simulink model "quad"  (R2022a)
settings: Solver=VariableStepAuto  StartTime=0.0  StopTime=5  RelTol=1e-3
values from neighbouring files (symbols this model uses):
  kp_yaw = omega_n_yaw^2*Izc    (= 0.0175335533676)    [ParamsInit_test.m]
undefined symbols (not defined in the file or in its folder): kp_height, kp_pitch, kp_roll, ModelInit_RPM, ModelParam_motorT, Newton, Raphson, stateInp, Timestep, Vehicle
libraries: simulink_extras x3, shared6dof x1
settings Model: Creator=Admin  LastModifiedBy=gaowe
settings SolverCC: AlgebraicLoopSolver=TrustRegion
settings DebuggingCC: UnconnectedInputMsg=warning  UnconnectedOutputMsg=warning  UnconnectedLineMsg=warning
settings RTWCC: DLArmComputeVersion=19.05

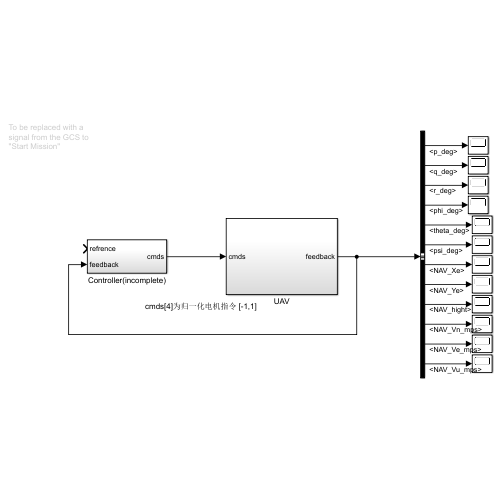
[thumbnail: Simulink's stored preview of the top-level diagram]
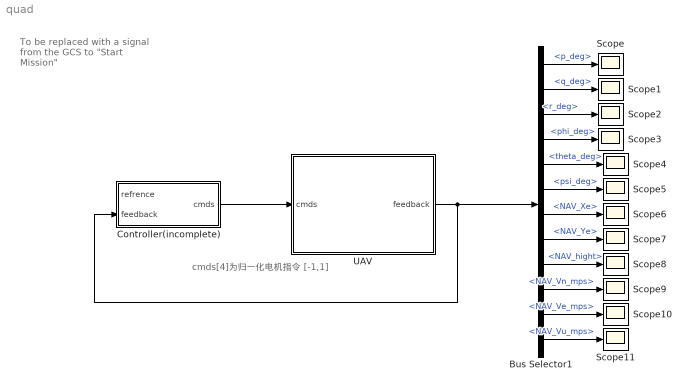
== system quad ==
  note: cmds[4]为归一化电机指令 [-1,1]
  note: To be replaced with a signal from the GCS to "Start Mission"
  Bus Selector1 : BusSelector  OutputSignals=MAG3.p_deg,MAG3.q_deg,MAG3.r_deg,MIDG.phi_deg,MIDG.theta_deg,MIDG.psi_deg,MIDG.NAV_Xe,MIDG.NAV_Ye,MIDG.NAV_hight,MIDG.NAV_Vn_mps,MIDG.NAV_Ve_mps,MIDG.NAV_Vu_mps
  Controller(incomplete) : Subsystem
  Scope{,1..11} (12 alike) : Scope
  UAV : Subsystem
  wires:
  Controller(incomplete)/1(cmds) -> UAV/1(cmds)
  UAV/1(feedback) -> Controller(incomplete)/2(feedback), Bus Selector1/1
  Bus Selector1/1 -> Scope/1  "<p_deg>"
  Bus Selector1/2 -> Scope1/1  "<q_deg>"
  Bus Selector1/3 -> Scope2/1  "<r_deg>"
  Bus Selector1/4 -> Scope3/1  "<phi_deg>"
  Bus Selector1/5 -> Scope4/1  "<theta_deg>"
  Bus Selector1/6 -> Scope5/1  "<psi_deg>"
  Bus Selector1/7 -> Scope6/1  "<NAV_Xe>"
  Bus Selector1/8 -> Scope7/1  "<NAV_Ye>"
  Bus Selector1/9 -> Scope8/1  "<NAV_hight>"
  Bus Selector1/10 -> Scope9/1  "<NAV_Vn_mps>"
  Bus Selector1/11 -> Scope10/1  "<NAV_Ve_mps>"
  Bus Selector1/12 -> Scope11/1  "<NAV_Vu_mps>"

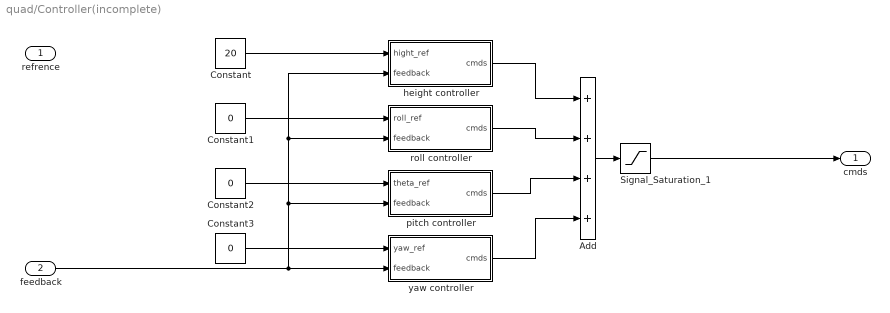
== system quad/Controller(incomplete) ==
  refrence : Inport
  feedback : Inport  Port=2
  Add : Sum  Inputs=++++
  Constant : Constant  Value=20
  Constant1 : Constant  Value=0
  Constant2 : Constant  Value=0
  Constant3 : Constant  Value=0
  Signal_Saturation_1 : Saturate  UpperLimit=[1 1 1 1]  LowerLimit=[-1 -1 -1 -1]
  height controller : Subsystem
  pitch controller : Subsystem
  roll controller : Subsystem
  yaw controller : Subsystem
  cmds : Outport
  wires:
  feedback/1 -> yaw controller/2(feedback), height controller/2(feedback), roll controller/2(feedback), pitch controller/2(feedback)
  Constant/1 -> height controller/1(hight_ref)
  Constant1/1 -> roll controller/1(roll_ref)
  roll controller/1(cmds) -> Add/2
  pitch controller/1(cmds) -> Add/3
  yaw controller/1(cmds) -> Add/4
  height controller/1(cmds) -> Add/1
  Add/1 -> Signal_Saturation_1/1
  Constant2/1 -> pitch controller/1(theta_ref)
  Constant3/1 -> yaw controller/1(yaw_ref)
  Signal_Saturation_1/1 -> cmds/1

== system quad/UAV ==
  cmds : Inport
  FM : Subsystem
  Sensors : Subsystem
  UAV Model : Subsystem
  feedback : Outport
  wires:
  UAV Model/2(Aux_Vars) -> Sensors/2(Aux_Vars), FM/3(Aux_Vars)
  FM/1(F_cg) -> UAV Model/1(Forces)
  FM/2(M_cg) -> UAV Model/2(Moments)
  UAV Model/1(EOM_States) -> Sensors/1(EOM_States), FM/2(EOM_States)
  Sensors/1(sensors) -> feedback/1
  cmds/1 -> FM/1(cmds)

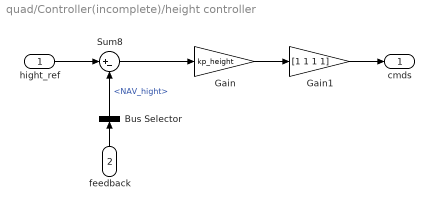
== system quad/Controller(incomplete)/height controller ==
  hight_ref : Inport
  feedback : Inport  Port=2
  Bus Selector : BusSelector  OutputSignals=MIDG.NAV_hight
  Gain : Gain  Gain=kp_height
  Gain1 : Gain  Gain=[1 1 1 1]
  Sum8 : Sum  Inputs=|+-
  cmds : Outport  VectorParamsAs1DForOutWhenUnconnected=off
  wires:
  hight_ref/1 -> Sum8/1
  feedback/1 -> Bus Selector/1
  Sum8/1 -> Gain/1
  Gain/1 -> Gain1/1
  Bus Selector/1 -> Sum8/2  "<NAV_hight>"
  Gain1/1 -> cmds/1

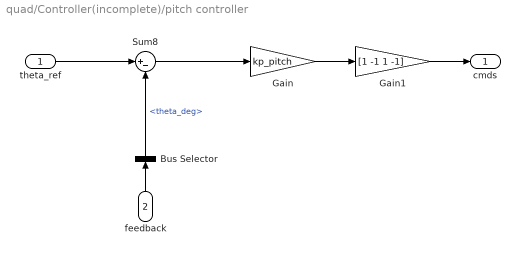
== system quad/Controller(incomplete)/pitch controller ==
  theta_ref : Inport
  feedback : Inport  Port=2
  Bus Selector : BusSelector  OutputSignals=MIDG.theta_deg
  Gain : Gain  Gain=kp_pitch
  Gain1 : Gain  Gain=[1 -1 1 -1]
  Sum8 : Sum  Inputs=|+-
  cmds : Outport  VectorParamsAs1DForOutWhenUnconnected=off
  wires:
  feedback/1 -> Bus Selector/1
  Sum8/1 -> Gain/1
  theta_ref/1 -> Sum8/1
  Gain/1 -> Gain1/1
  Bus Selector/1 -> Sum8/2  "<theta_deg>"
  Gain1/1 -> cmds/1

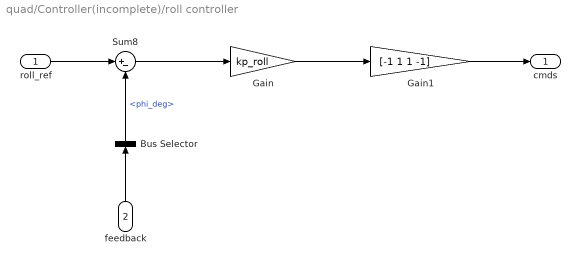
== system quad/Controller(incomplete)/roll controller ==
  roll_ref : Inport
  feedback : Inport  Port=2
  Bus Selector : BusSelector  OutputSignals=MIDG.phi_deg
  Gain : Gain  Gain=kp_roll
  Gain1 : Gain  Gain=[-1 1 1 -1]
  Sum8 : Sum  Inputs=|+-
  cmds : Outport  VectorParamsAs1DForOutWhenUnconnected=off
  wires:
  roll_ref/1 -> Sum8/1
  Sum8/1 -> Gain/1
  feedback/1 -> Bus Selector/1
  Gain/1 -> Gain1/1
  Bus Selector/1 -> Sum8/2  "<phi_deg>"
  Gain1/1 -> cmds/1

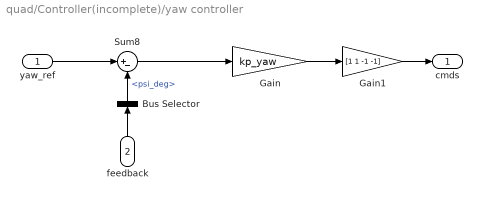
== system quad/Controller(incomplete)/yaw controller ==
  yaw_ref : Inport
  feedback : Inport  Port=2
  Bus Selector : BusSelector  OutputSignals=MIDG.psi_deg
  Gain : Gain  Gain=kp_yaw
  Gain1 : Gain  Gain=[1 1 -1 -1]
  Sum8 : Sum  Inputs=|+-
  cmds : Outport  VectorParamsAs1DForOutWhenUnconnected=off
  wires:
  feedback/1 -> Bus Selector/1
  Sum8/1 -> Gain/1
  yaw_ref/1 -> Sum8/1
  Gain/1 -> Gain1/1
  Bus Selector/1 -> Sum8/2  "<psi_deg>"
  Gain1/1 -> cmds/1

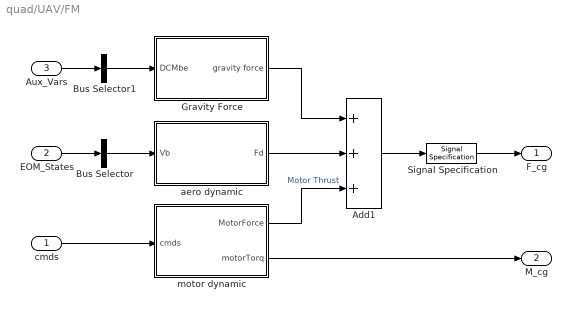
== system quad/UAV/FM ==
  cmds : Inport
  EOM_States : Inport  Port=2  Unit=m/s
  Aux_Vars : Inport  Port=3
  Add1 : Sum  Inputs=+++
  Bus Selector : BusSelector  OutputSignals=ub,wb,vb  OutputAsBus=on
  Bus Selector1 : BusSelector  OutputSignals=DCMbe  OutputAsBus=on
  Gravity Force : Subsystem
  Signal Specification : SignalSpecification  Dimensions=3
  aero dynamic : Subsystem
  motor dynamic : Subsystem
  F_cg : Outport  Unit=N  VectorParamsAs1DForOutWhenUnconnected=off
  M_cg : Outport  Port=2  Unit=N*m  VectorParamsAs1DForOutWhenUnconnected=off
  wires:
  Signal Specification/1 -> F_cg/1
  Aux_Vars/1 -> Bus Selector1/1
  cmds/1 -> motor dynamic/1(cmds)
  motor dynamic/2(motorTorq) -> M_cg/1
  Add1/1 -> Signal Specification/1
  Gravity Force/1(gravity force) -> Add1/1
  motor dynamic/1(MotorForce) -> Add1/3  "Motor Thrust"
  EOM_States/1 -> Bus Selector/1
  aero dynamic/1(Fd) -> Add1/2
  Bus Selector/1 -> aero dynamic/1(Vb)
  Bus Selector1/1 -> Gravity Force/1(DCMbe)

== system quad/UAV/Sensors ==
  EOM_States : Inport
  Aux_Vars : Inport  Port=2
  Bus Creator1 : BusCreator  Inputs=2
  MAG3 IMU : Subsystem
  MIDG II 50 Hz : Subsystem  SystemSampleTime=round(1/Timestep/50)*Timestep
  sensors : Outport
  wires:
  Bus Creator1/1 -> sensors/1
  MIDG II 50 Hz/1(MIDG) -> Bus Creator1/1  "MIDG"
  MAG3 IMU/1(MAG3) -> Bus Creator1/2  "MAG3"
  Aux_Vars/1 -> MIDG II 50 Hz/2(AuxVars)
  EOM_States/1 -> MAG3 IMU/1(EOM_State), MIDG II 50 Hz/1(EOM_State)

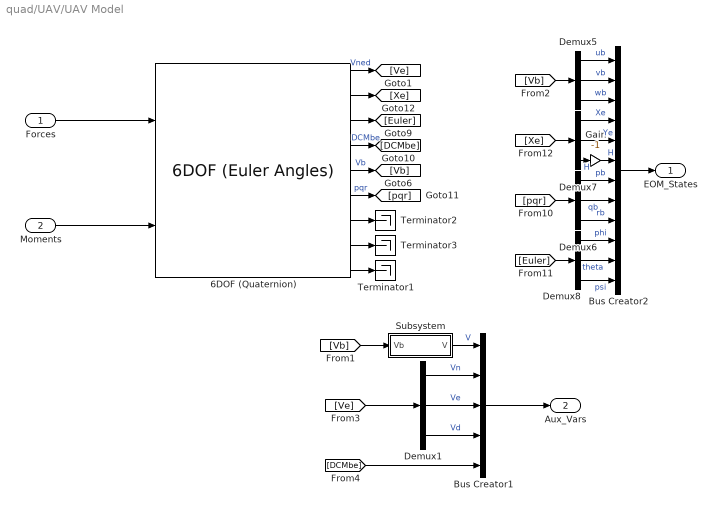
== system quad/UAV/UAV Model ==
  Forces : Inport
  Moments : Inport  Port=2
  6DOF (Quaternion) : shared6dof/6DOF (Euler Angles)  units=Metric (MKS)  mtype=Fixed  rep=Euler Angles  xme_0=stateInp.xyz.*[1 1 -1]  Vm_0=stateInp.uvw  eul_0=stateInp.euler  pm_0=stateInp.pqr  mass_0=Vehicle.Airframe.mass  mass_e=0.5  mass_f=2.0  inertia=Vehicle.Airfame.inertia  inertia_e=eye(3)  inertia_f=2*eye(3)  k_quat=Vehicle.SixDOF.quatGain  vre_flag=on  abi_flag=on  aMode=aMode  xme_statename=''  Vm_statename=''  eul_statename=''  quat_statename=''  pm_statename=''  mass_statename=''
      settings: SourceProductBaseCode=AE,PW,DR,MT,VE
  Bus Creator1 : BusCreator  Inputs=5
  Bus Creator2 : BusCreator  Inputs=12
  Demux{1,5..8} (5 alike) : Demux  Outputs=3
  Gain : Gain  Gain=-1
  Subsystem : Subsystem
  Terminator1 : Terminator
  Terminator2 : Terminator
  Terminator3 : Terminator
  EOM_States : Outport
  Aux_Vars : Outport  Port=2
  wires:
  Moments/1 -> 6DOF (Quaternion)/2
  6DOF (Quaternion)/8 -> Terminator3/1
  6DOF (Quaternion)/7 -> Terminator2/1
  6DOF (Quaternion)/9 -> Terminator1/1
  Forces/1 -> 6DOF (Quaternion)/1
  Demux8/2 -> Bus Creator2/11  "theta"
  [Euler] -> Demux8/1
  [Vb] -> Demux5/1
  Bus Creator2/1 -> EOM_States/1
  [pqr] -> Demux6/1
  Demux6/3 -> Bus Creator2/9  "rb"
  Demux7/1 -> Bus Creator2/4  "Xe"
  [Xe] -> Demux7/1
  Demux7/2 -> Bus Creator2/5  "Ye"
  Demux5/1 -> Bus Creator2/1  "ub"
  Demux6/1 -> Bus Creator2/7  "pb"
  Demux5/2 -> Bus Creator2/2  "vb"
  Demux8/3 -> Bus Creator2/12  "psi"
  Demux7/3 -> Gain/1  "H"
  Demux5/3 -> Bus Creator2/3  "wb"
  Demux8/1 -> Bus Creator2/10  "phi"
  Demux6/2 -> Bus Creator2/8  "qb"
  6DOF (Quaternion)/2 -> [Xe]
  6DOF (Quaternion)/3 -> [Euler]
  6DOF (Quaternion)/4 -> [DCMbe]  "DCMbe"
  6DOF (Quaternion)/5 -> [Vb]  "Vb"
  6DOF (Quaternion)/6 -> [pqr]  "pqr"
  6DOF (Quaternion)/1 -> [Ve]  "Vned"
  Bus Creator1/1 -> Aux_Vars/1
  Subsystem/1(V) -> Bus Creator1/1  "V"
  [Vb] -> Subsystem/1(Vb)
  Demux1/1 -> Bus Creator1/2  "Vn"
  Demux1/2 -> Bus Creator1/3  "Ve"
  Demux1/3 -> Bus Creator1/4  "Vd"
  [Ve] -> Demux1/1
  Gain/1 -> Bus Creator2/6  "H"
  [DCMbe] -> Bus Creator1/5

== system quad/UAV/FM/Gravity Force ==
  DCMbe : Inport
  D2 : Constant  Value=[0 0 9.8]
  Gain1 : Gain  Gain=Vehicle.Airframe.mass
  Product : Product  Multiplication=Matrix(*)
  gravity force : Outport  Unit=N  VectorParamsAs1DForOutWhenUnconnected=off
  wires:
  D2/1 -> Gain1/1
  Gain1/1 -> Product/2  "gravity force NED"
  Product/1 -> gravity force/1
  DCMbe/1 -> Product/1

== system quad/UAV/FM/aero dynamic ==
  Vb : Inport
  Cd : Constant  Value=0.073
  Fd Calculate : MATLAB Function  TreatAsAtomicUnit=on
  Fd : Outport
  wires:
  Cd/1 -> Fd Calculate/2(Cd)
  Fd Calculate/1(Fd) -> Fd/1
  Vb/1 -> Fd Calculate/1(Vb)

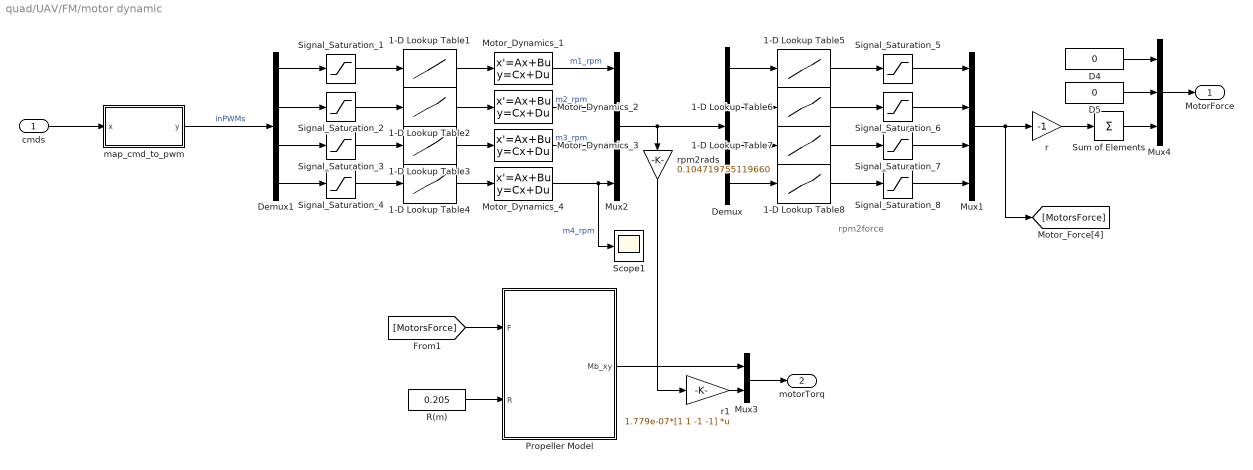
== system quad/UAV/FM/motor dynamic ==
  note: rpm2force
  cmds : Inport
  1-D Lookup Table1 : Lookup_n-D  NumberOfTableDimensions=1  BreakpointsForDimension1=|  BeginIndexSearchUsingPreviousIndexResult=on  Table=|  InternalRulePriority=Speed  RndMeth=Simplest
      BreakpointsForDimension1=|
      | [1301
      | 1347
      | 1402
      | 1459
      | 1522
      | 1591
      | 1661
      | 1702
      | 1778
      | 1932]
      Table=|
      | [2847
      | 3689
      | 4585
      | 5400
      | 6400
      | 7000
      | 7800
      | 8222
      | 9300
      | 10700]
  1-D Lookup Table2 : Lookup_n-D  NumberOfTableDimensions=1  BreakpointsForDimension1=|  BeginIndexSearchUsingPreviousIndexResult=on  Table=|  InternalRulePriority=Speed  RndMeth=Simplest
      BreakpointsForDimension1=|
      | [1301
      | 1347
      | 1402
      | 1459
      | 1522
      | 1591
      | 1661
      | 1702
      | 1778
      | 1932]
      Table=|
      | [2847
      | 3689
      | 4585
      | 5400
      | 6400
      | 7000
      | 7800
      | 8222
      | 9300
      | 10700]
  1-D Lookup Table3 : Lookup_n-D  NumberOfTableDimensions=1  BreakpointsForDimension1=|  BeginIndexSearchUsingPreviousIndexResult=on  Table=|  InternalRulePriority=Speed  RndMeth=Simplest
      BreakpointsForDimension1=|
      | [1301
      | 1347
      | 1402
      | 1459
      | 1522
      | 1591
      | 1661
      | 1702
      | 1778
      | 1932]
      Table=|
      | [2847
      | 3689
      | 4585
      | 5400
      | 6400
      | 7000
      | 7800
      | 8222
      | 9300
      | 10700]
  1-D Lookup Table4 : Lookup_n-D  NumberOfTableDimensions=1  BreakpointsForDimension1=|  BeginIndexSearchUsingPreviousIndexResult=on  Table=|  InternalRulePriority=Speed  RndMeth=Simplest
      BreakpointsForDimension1=|
      | [1301
      | 1347
      | 1402
      | 1459
      | 1522
      | 1591
      | 1661
      | 1702
      | 1778
      | 1932]
      Table=|
      | [2847
      | 3689
      | 4585
      | 5400
      | 6400
      | 7000
      | 7800
      | 8222
      | 9300
      | 10700]
  1-D Lookup Table5 : Lookup_n-D  NumberOfTableDimensions=1  BreakpointsForDimension1=|  BeginIndexSearchUsingPreviousIndexResult=on  Table=|  InternalRulePriority=Speed  RndMeth=Simplest
      BreakpointsForDimension1=|
      | [2847
      | 3689
      | 4585
      | 5400
      | 6400
      | 7000
      | 7800
      | 8222
      | 9300
      | 10700]
      Table=|
      | [0.6664
      | 1.4308
      | 2.3422
      | 3.3418
      | 4.9098
      | 5.929
      | 7.399
      | 7.6244
      | 10.976
      | 13.72]
  1-D Lookup Table6 : Lookup_n-D  NumberOfTableDimensions=1  BreakpointsForDimension1=|  BeginIndexSearchUsingPreviousIndexResult=on  Table=|  InternalRulePriority=Speed  RndMeth=Simplest
      BreakpointsForDimension1=|
      | [2847
      | 3689
      | 4585
      | 5400
      | 6400
      | 7000
      | 7800
      | 8222
      | 9300
      | 10700]
      Table=|
      | [0.6664
      | 1.4308
      | 2.3422
      | 3.3418
      | 4.9098
      | 5.929
      | 7.399
      | 7.6244
      | 10.976
      | 13.72]
  1-D Lookup Table7 : Lookup_n-D  NumberOfTableDimensions=1  BreakpointsForDimension1=|  BeginIndexSearchUsingPreviousIndexResult=on  Table=|  InternalRulePriority=Speed  RndMeth=Simplest
      BreakpointsForDimension1=|
      | [2847
      | 3689
      | 4585
      | 5400
      | 6400
      | 7000
      | 7800
      | 8222
      | 9300
      | 10700]
      Table=|
      | [0.6664
      | 1.4308
      | 2.3422
      | 3.3418
      | 4.9098
      | 5.929
      | 7.399
      | 7.6244
      | 10.976
      | 13.72]
  1-D Lookup Table8 : Lookup_n-D  NumberOfTableDimensions=1  BreakpointsForDimension1=|  BeginIndexSearchUsingPreviousIndexResult=on  Table=|  InternalRulePriority=Speed  RndMeth=Simplest
      BreakpointsForDimension1=|
      | [2847
      | 3689
      | 4585
      | 5400
      | 6400
      | 7000
      | 7800
      | 8222
      | 9300
      | 10700]
      Table=|
      | [0.6664
      | 1.4308
      | 2.3422
      | 3.3418
      | 4.9098
      | 5.929
      | 7.399
      | 7.6244
      | 10.976
      | 13.72]
  D4 : Constant  Value=0
  D5 : Constant  Value=0
  Demux : Demux
  Demux1 : Demux
  Motor_Dynamics_{1..4} (4 alike) : StateSpace  A=-1/ModelParam_motorT  C=1/ModelParam_motorT  D=0  InitialCondition=ModelInit_RPM*ModelParam_motorT
  Mux1 : Mux
  Mux2 : Mux
  Mux3 : Mux  Inputs=[2 1]
  Mux4 : Mux  Inputs=3
  Propeller Model : MATLAB Function  TreatAsAtomicUnit=on
  R(m) : Constant  Value=0.205
  Scope1 : Scope
  Signal_Saturation_{1..4} (4 alike) : Saturate  UpperLimit=2400  LowerLimit=0
  Signal_Saturation_{5..8} (4 alike) : Saturate  UpperLimit=1.4*9.8  LowerLimit=0
  Sum of Elements : Sum  Inputs=+
  map_cmd_to_pwm : Subsystem  AncestorBlock=neural/Processing Functions/mapminmax  mask(MAPMINMAX Preprocess){xmin=[-1 -1 -1 -1], xmax=[1 1 1 1], ymin=[1000 1000 1000 1000], ymax=[2000 2000 2000 2000]}
      mask prompts: xmin "Minimum X (Nx1 column)"; xmax "Maximum X (Nx1 column)"; ymin "Minimum Y"; ymax "Maximum Y"
      mask help: Maps each element of x from its respective [minimum,maximum] interval to a common [minimum,maximum] interval.
      mask init:
      | network;
      mask Help: helpview([docroot '/deeplearning/ref/mapminmax.html']);
      mask Display:
      | e = 0.06;
      | c1 = [120 150 230]/255;
      | c2 = ([120 150 230]+0)/383;
      | c3 = ([120 150 230]+128)/383;
      | patch([0 1 1 0],[0 0 1 1],c1);
      | patch([0 1 1 1-e 1-e 0+e],[0 0 1 1-e 0+e 0+e],c2);
      | patch([0 0 1 1-e 0+e 0+e],[0 1 1 1-e 1-e 0+e],c3);
      | plot([0 1 1 0 0],[0 0 1 1 0])
      | port_label('input',1,'x')
      | port_label('output',1,'y')
  r : Gain  Gain=-1
  r1 : Gain  Gain=1.779e-07*[1 1 -1 -1]  Multiplication=Matrix(K*u)
  rpm2rads : Gain  Gain=0.104719755119660
  MotorForce : Outport
  motorTorq : Outport  Port=2
  wires:
  Demux1/2 -> Signal_Saturation_2/1
  Signal_Saturation_2/1 -> 1-D Lookup Table2/1
  Demux1/1 -> Signal_Saturation_1/1
  Signal_Saturation_1/1 -> 1-D Lookup Table1/1
  Demux1/3 -> Signal_Saturation_3/1
  1-D Lookup Table1/1 -> Motor_Dynamics_1/1
  1-D Lookup Table2/1 -> Motor_Dynamics_2/1
  Signal_Saturation_3/1 -> 1-D Lookup Table3/1
  Signal_Saturation_4/1 -> 1-D Lookup Table4/1
  Demux1/4 -> Signal_Saturation_4/1
  1-D Lookup Table4/1 -> Motor_Dynamics_4/1
  1-D Lookup Table3/1 -> Motor_Dynamics_3/1
  1-D Lookup Table5/1 -> Signal_Saturation_5/1
  1-D Lookup Table6/1 -> Signal_Saturation_6/1
  1-D Lookup Table7/1 -> Signal_Saturation_7/1
  1-D Lookup Table8/1 -> Signal_Saturation_8/1
  Signal_Saturation_5/1 -> Mux1/1
  Signal_Saturation_6/1 -> Mux1/2
  Signal_Saturation_7/1 -> Mux1/3
  Signal_Saturation_8/1 -> Mux1/4
  rpm2rads/1 -> r1/1
  Mux2/1 -> Demux/1, rpm2rads/1
  R(m)/1 -> Propeller Model/2(R)
  Propeller Model/1(Mb_xy) -> Mux3/1
  Mux3/1 -> motorTorq/1
  r/1 -> Sum of Elements/1
  D4/1 -> Mux4/1
  D5/1 -> Mux4/2
  Mux4/1 -> MotorForce/1
  r1/1 -> Mux3/2
  Mux1/1 -> [MotorsForce], r/1
  cmds/1 -> map_cmd_to_pwm/1(x)
  Motor_Dynamics_1/1 -> Mux2/1  "m1_rpm"
  Motor_Dynamics_2/1 -> Mux2/2  "m2_rpm"
  Motor_Dynamics_3/1 -> Mux2/3  "m3_rpm"
  Motor_Dynamics_4/1 -> Scope1/1, Mux2/4  "m4_rpm"
  Demux/4 -> 1-D Lookup Table8/1
  Demux/3 -> 1-D Lookup Table7/1
  Demux/2 -> 1-D Lookup Table6/1
  Demux/1 -> 1-D Lookup Table5/1
  [MotorsForce] -> Propeller Model/1(F)
  map_cmd_to_pwm/1(y) -> Demux1/1  "inPWMs"
  Sum of Elements/1 -> Mux4/3

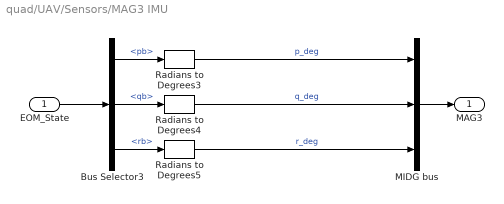
== system quad/UAV/Sensors/MAG3 IMU ==
  EOM_State : Inport
  Bus Selector3 : BusSelector  OutputSignals=pb,qb,rb
  MIDG bus : BusCreator  Inputs=3
  Radians to Degrees3 : simulink_extras/Transformations/Radians to Degrees
  Radians to Degrees4 : simulink_extras/Transformations/Radians to Degrees
  Radians to Degrees5 : simulink_extras/Transformations/Radians to Degrees
  MAG3 : Outport
  wires:
  Radians to Degrees5/1 -> MIDG bus/3  "r_deg"
  Radians to Degrees4/1 -> MIDG bus/2  "q_deg"
  Radians to Degrees3/1 -> MIDG bus/1  "p_deg"
  EOM_State/1 -> Bus Selector3/1
  Bus Selector3/1 -> Radians to Degrees3/1  "<pb>"
  Bus Selector3/2 -> Radians to Degrees4/1  "<qb>"
  Bus Selector3/3 -> Radians to Degrees5/1  "<rb>"
  MIDG bus/1 -> MAG3/1

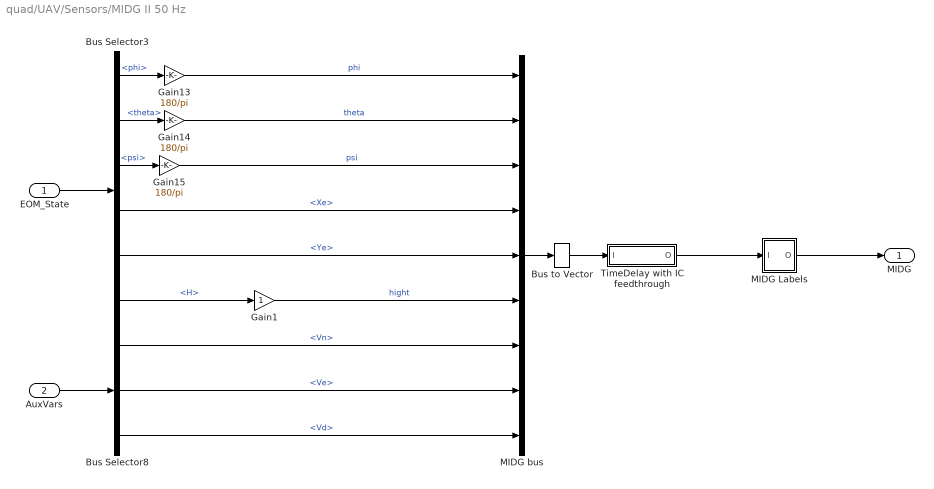
== system quad/UAV/Sensors/MIDG II 50 Hz ==
  EOM_State : Inport
  AuxVars : Inport  Port=2
  Bus Selector3 : BusSelector  OutputSignals=phi,theta,psi,Xe,Ye,H
  Bus Selector8 : BusSelector  OutputSignals=Vn,Ve,Vd
  Bus to Vector : BusToVector
  Gain1 : Gain
  Gain13 : Gain  Gain=180/pi
  Gain14 : Gain  Gain=180/pi
  Gain15 : Gain  Gain=180/pi
  MIDG Labels : Subsystem
  MIDG bus : BusCreator  Inputs=9
  TimeDelay with IC feedthrough : Subsystem  mask{TimeDelay=40e-3}
      mask prompts: TimeDelay "Time Delay (sec)"
      mask help:
      | Implements Continuous Time Transport Delay with initial
      | outputs set to feedthrough with no delay.
      |
      |   output = input;   for t<TimeDelay
      |   output = input(t-tdelay); for t>=TimeDelay
  MIDG : Outport
  wires:
  Bus to Vector/1 -> TimeDelay with IC feedthrough/1(I)
  MIDG bus/1 -> Bus to Vector/1
  EOM_State/1 -> Bus Selector3/1
  Bus Selector3/1 -> Gain13/1  "<phi>"
  Bus Selector3/2 -> Gain14/1  "<theta>"
  Bus Selector3/3 -> Gain15/1  "<psi>"
  Gain13/1 -> MIDG bus/1  "phi"
  Gain14/1 -> MIDG bus/2  "theta"
  Gain15/1 -> MIDG bus/3  "psi"
  Gain1/1 -> MIDG bus/6  "hight"
  Bus Selector3/4 -> MIDG bus/4  "<Xe>"
  Bus Selector3/5 -> MIDG bus/5  "<Ye>"
  Bus Selector3/6 -> Gain1/1  "<H>"
  MIDG Labels/1(O) -> MIDG/1
  TimeDelay with IC feedthrough/1(O) -> MIDG Labels/1(I)
  AuxVars/1 -> Bus Selector8/1
  Bus Selector8/3 -> MIDG bus/9  "<Vd>"
  Bus Selector8/2 -> MIDG bus/8  "<Ve>"
  Bus Selector8/1 -> MIDG bus/7  "<Vn>"

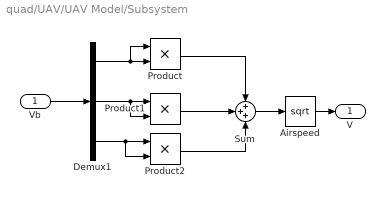
== system quad/UAV/UAV Model/Subsystem ==
  Vb : Inport
  Airspeed : Sqrt  AlgorithmType=Newton-Raphson
  Demux1 : Demux  Outputs=3
  Product : Product  RndMeth=Zero
  Product1 : Product  RndMeth=Zero
  Product2 : Product  RndMeth=Zero
  Sum : Sum  Inputs=+++
  V : Outport
  wires:
  Airspeed/1 -> V/1
  Sum/1 -> Airspeed/1
  Demux1/2 -> Product1/1, Product1/2
  Demux1/3 -> Product2/2, Product2/1
  Product/1 -> Sum/1
  Product2/1 -> Sum/3
  Demux1/1 -> Product/2, Product/1
  Product1/1 -> Sum/2
  Vb/1 -> Demux1/1

== system quad/UAV/FM/motor dynamic/map_cmd_to_pwm ==
  x : Inport
  Add min y : Bias  Bias=ymin  SaturateOnIntegerOverflow=off
  Subtract min x : Bias  Bias=-xmin  SaturateOnIntegerOverflow=off
  range y / range x : Gain  Gain=(ymax-ymin)./(xmax-xmin)
  y : Outport  VectorParamsAs1DForOutWhenUnconnected=off
  wires:
  Add min y/1 -> y/1
  range y / range x/1 -> Add min y/1
  Subtract min x/1 -> range y / range x/1
  x/1 -> Subtract min x/1

== system quad/UAV/Sensors/MIDG II 50 Hz/MIDG Labels ==
  I : Inport
  Bus Creator : BusCreator  Inputs=9
  Demux : Demux  Outputs=9
  O : Outport
  wires:
  I/1 -> Demux/1
  Bus Creator/1 -> O/1
  Demux/2 -> Bus Creator/2  "theta_deg"
  Demux/1 -> Bus Creator/1  "phi_deg"
  Demux/4 -> Bus Creator/4  "NAV_Xe"
  Demux/5 -> Bus Creator/5  "NAV_Ye"
  Demux/6 -> Bus Creator/6  "NAV_hight"
  Demux/7 -> Bus Creator/7  "NAV_Vn_mps"
  Demux/8 -> Bus Creator/8  "NAV_Ve_mps"
  Demux/9 -> Bus Creator/9  "NAV_Vu_mps"
  Demux/3 -> Bus Creator/3  "psi_deg"

== system quad/UAV/Sensors/MIDG II 50 Hz/TimeDelay with IC feedthrough ==
  I : Inport
  Clock : Clock
  Switch : Switch  Criteria=u2 > Threshold  Threshold=TimeDelay  SaturateOnIntegerOverflow=off  InputSameDT=off
  Transport Delay : TransportDelay  DelayTime=TimeDelay
      settings: AttributesFormatString=%<DelayTime>
  O : Outport
  wires:
  I/1 -> Transport Delay/1, Switch/3
  Clock/1 -> Switch/2
  Switch/1 -> O/1
  Transport Delay/1 -> Switch/1

== matlab function quad/UAV/FM/aero dynamic/Fd Calculate ==
  data: Fd output; Vb input; Cd input
function Fd  = fcn(Vb,Cd)
 %%叉字型
 %3  1
 %2  4
 Fd = -Cd*Vb.*abs(Vb)*0.5;
end

== matlab function quad/UAV/FM/motor dynamic/Propeller Model ==
  data: Mb_xy output; F input; R input
function Mb_xy  = fcn(F,R)
 %%叉字型
 %3  1
 %2  4
 M_rctcm = [-sin(pi/4)*R,sin(pi/4)*R,sin(pi/4)*R,-sin(pi/4)*R;
            sin(pi/4)*R,-sin(pi/4)*R,sin(pi/4)*R,-sin(pi/4)*R];
 Mb_xy = M_rctcm*(F);%式(6.24),力矩

end
